simulink model "untitled1"  (R2014b)
settings: Solver=ode45  StartTime=0.0  StopTime=0.02  RelTol=1e-3
undefined symbols (not defined in the file or in its folder): powergui
libraries: powerlib x11
settings Model: Creator=JPSOLIV  LastModifiedBy=JPSOLIV

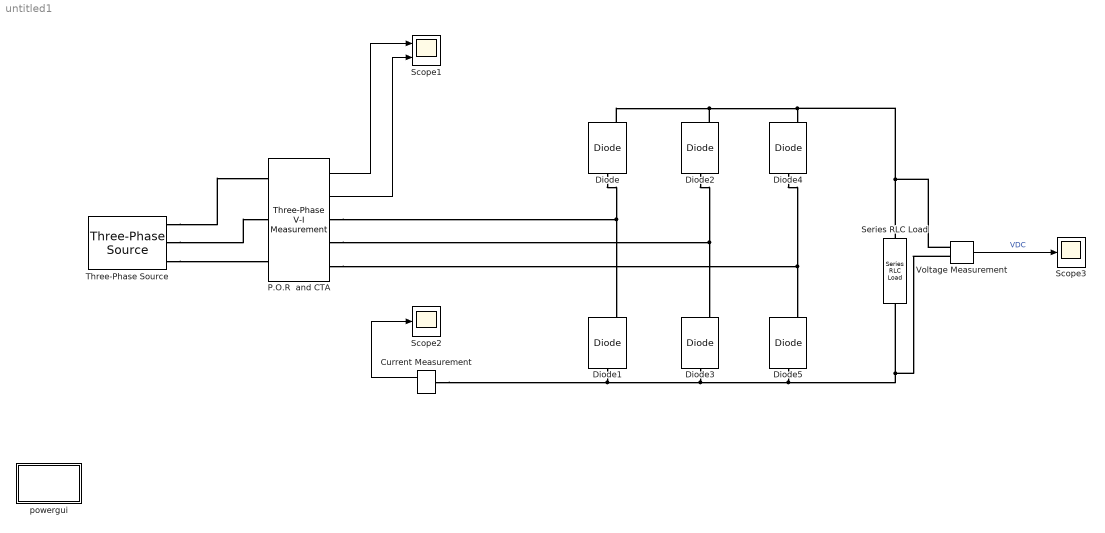
== system untitled1 ==
  Current Measurement : powerlib/Measurements/Current Measurement  PhasorSimulation=off  OutputType=Complex  PSBequivalent=0
  Diode{,1..5} (6 alike) : powerlib/Power Electronics/Diode  Ron=0.001  Lon=0  Vf=0.8  IC=0  UseSnubber=off  Rs=500  Cs=250e-9  Measurements=on
  P.O.R  and CTA : powerlib/Measurements/Three-Phase V-I Measurement  VoltageMeasurement=phase-to-phase  SetLabelV=off  LabelV=Vabc  Vpu=off  VpuLL=off  CurrentMeasurement=yes  SetLabelI=off  LabelI=Iabc  Ipu=off  Pbase=100e6  Vbase=500e3  OutputType=Complex  PhasorSimulation=off  PSBequivalent=0
  Scope1 : Scope  NumInputPorts=2
      settings: TimeRange=0.005  YMin=-200~-5  YMax=200~5  Decimation=100  SampleTime=1e-3
  Scope2 : Scope
      settings: TimeRange=0.005  YMin=-200  YMax=200  Decimation=100  SampleTime=1e-3
  Scope3 : Scope
      settings: TimeRange=0.005  YMin=-200  YMax=200  SaveName=ScopeData2  Decimation=100  SampleTime=1e-3
  Series RLC Load : powerlib/Elements/Series RLC Load  LConnTagsString=a  RConnTagsString=__new0  NominalVoltage=280  NominalFrequency=400  ActivePower=200  InductivePower=100  CapacitivePower=0  Setx0=off  InitialVoltage=0  SetiL0=off  InitialCurrent=0  Measurements=None
  Three-Phase Source : powerlib/Electrical Sources/Three-Phase Source  Voltage=115*sqrt(3)  PhaseAngle=0  Frequency=400  InternalConnection=Yn  SpecifyImpedance=off  Resistance=0.8929e-6  Inductance=16.58e-3*1e-6  ShortCircuitLevel=100e6  BaseVoltage=25e3  XRratio=7  BusType=swing  Pref=0  Qref=0  Qmin=-inf  Qmax=inf
  Voltage Measurement : powerlib/Measurements/Voltage Measurement  PhasorSimulation=off  OutputType=Complex  PSBequivalent=0
  powergui : Subsystem  Priority=1  AncestorBlock=powerlib/powergui  InitFcn=powergui( 'InitFcn_Callback' , gcb , 0 , [ ] );  StopFcn=powergui( 'StopFcn_Callback' , gcb , 0 , [ ] );  mask(PSB option menu block){SimulationMode=Discrete, SolverType=Tustin, SampleTime=1e-7, frequency=60, SPID=off, DisableSnubberDevices=off, DisableRonSwitches=off, DisableVfSwitches=off, SwTol=0, DisplayEquations=off, Interpol=off, methode=off, Ts=0, frequencyindice=0, Pbase=100e6, ErrMax=1e-4, Iterations=50, UnitsV=kV, UnitsW=MW, FunctionMessages=off, echomessages=off, HookPort=off, EnableUseOfTLC=off, x0status=blocks, RestoreLinks=warning, ResistiveCurrentMeasurement=off, Frange=[0:2:500], Ylog=off, Xlog=on, ShowGrid=off, save=off, variable=ZData, structure=0, ZoomFFT=off, StartTime=0.0, cycles=1, DisplayStyle=1, fundamental=60, FreqAxis=off, MaxFrequency=1000, frequencyindicesteady=1, RmsSteady=1, display=off}
      mask prompts: SimulationMode "Simulation type:"; SolverType "Solver type:"; SampleTime "Sample time (s):"; frequency "Phasor frequency (Hz):"; SPID "Enable use of ideal switching devices"; DisableSnubberDevices "Disable snubbers in switching devices"; DisableRonSwitches "Disable On resistance in switching devices (Ron=0)"; DisableVfSwitches "Disable Forward voltage in switching devices (Vf=0)"; SwTol "Switch tolerance"; DisplayEquations "Display circuit differential equations"; Interpol "Interpolate"; methode "Store state-space matrices"; Ts "Buffer size (MBytes)"; frequencyindice "Load flow frequency (Hz):"; Pbase "Base power Pbase (VA):"; ErrMax "PQ tolerance (pu):"; Iterations "Max iterations:"; UnitsV "Voltage units"; UnitsW "Power units"; FunctionMessages "Disable SimPowerSystems warnings"; echomessages "Display SimPowerSystems compilation messages"; HookPort "Add a hook port to the powergui block"; EnableUseOfTLC "Use TLC file when in Accelerator Simulation Mode and for code generation"; x0status "Start simulation with initial electrical states from:"; RestoreLinks "Restore disabled links of SimPowerSystems blocks:"; ResistiveCurrentMeasurement "Use non ideal current measurement blocks (1e-4Ohm internal resistance)"; Frange "Frequency Range"; Ylog "Log impedance"; Xlog "log Frequency"; ShowGrid "grid"; save "Save Data To Workspace"; variable "Variable Name"; structure "Structure Name (PSBFFTSCOPE)"; ZoomFFT "ZoomFFT (PSBFFTSCOPE)"; StartTime "Start Time (PSBFFTSCOPE)"; cycles "Cycles (PSBFFTSCOPE)"; DisplayStyle "Display style (PSBFFTSCOPE)"; fundamental "Fundamental (PSBFFTSCOPE)"; FreqAxis "Frequency Axis (PSBFFTSCOPE)"; MaxFrequency "Max Frequency (PSBFFTSCOPE)"; frequencyindicesteady "Frequency indice (STEADYSTATE)"; RmsSteady "RMS display (STEADYSTATE)"; display "Display Results"
      mask help: Set simulation type, simulation parameters, and preferences
      mask init:
      | message = powergui('MaskInitialization',gcb,SimulationMode,SampleTime);
      settings: CopyFcn=powergui( 'Copy_Callback' , gcb , 0 , [ ] );  ModelCloseFcn=powergui( 'CloseButton_Callback' , gcb , [ ] , [ ] );  NameChangeFcn=powergui( 'NameChangeFcn_Callback' , gcb , 0 , [ ] );  OpenFcn=powergui(gcb,'Open')
      settings: DeleteFcn=|
      | % see geck 675031 powergui( 'Copy_Callback' , gcb , 1 , [ ] );
      | 
      | powergui( 'CloseButton_Callback' , gcb , [ ] , [ ] );
      settings: PreSaveFcn=|
      | powergui( 'PreSaveFcn_Callback' , gcb , [ ] , [ ] );
      | powergui( 'CloseButton_Callback' , gcb , [ ] , [ ] );
      mask Help: helpview(psbhelp)
      mask TypeOptions SimulationMode: Continuous | Discrete | Phasor
      mask Callback SimulationMode: powergui('SimulationType',[],[],gcb);
      mask TypeOptions SolverType: Tustin/Backward Euler (TBE) | Tustin | Backward Euler
      mask Callback SolverType: powergui('SolverType',[],[],gcb);
      mask Callback SPID: powergui('SPID',[],[],gcb);
      mask Callback Interpol: powergui('INTERPOLATE',[],[],gcb);
      mask Callback methode: powergui('STORE',[],[],gcb);
      mask TypeOptions UnitsV: V | kV
      mask TypeOptions UnitsW: W | kW | MW
      mask Callback HookPort: powergui('HookPort',[],[],gcb);
      mask TypeOptions x0status: blocks | steady | zero
      mask TypeOptions RestoreLinks: yes | warning | no
      mask DialogControl Advanced Prompt: Advanced settings (Tustin solver)
      mask Display: color('blue'),disp(message)
  wires:
  Voltage Measurement/1 -> Scope3/1  "VDC"
  P.O.R  and CTA/1 -> Scope1/1
  P.O.R  and CTA/2 -> Scope1/2
  Current Measurement/1 -> Scope2/1
  connections:
  Diode/LConn1 -- P.O.R  and CTA/RConn1 -- Diode1/RConn1
  Diode2/LConn1 -- P.O.R  and CTA/RConn2 -- Diode3/RConn1
  Diode4/RConn1 -- Diode/RConn1 -- Diode2/RConn1 -- Series RLC Load/LConn1 -- Voltage Measurement/LConn1
  Voltage Measurement/LConn2 -- Series RLC Load/RConn1 -- Diode5/LConn1 -- Current Measurement/LConn1 -- Diode1/LConn1 -- Diode3/LConn1
  Diode4/LConn1 -- P.O.R  and CTA/RConn3 -- Diode5/RConn1
  Three-Phase Source/RConn1 -- P.O.R  and CTA/LConn1
  Three-Phase Source/RConn2 -- P.O.R  and CTA/LConn2
  Three-Phase Source/RConn3 -- P.O.R  and CTA/LConn3

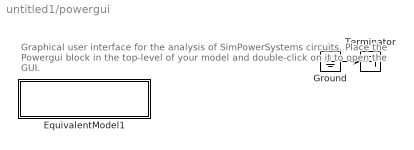
== system untitled1/powergui ==
  note: Graphical user interface for the analysis of  SimPowerSystems circuits.
      | Place the Powergui block in the top-level of your model and double-click
      | on it to open the GUI.
  EquivalentModel1 : Subsystem
      mask init:
      | S  = GetDataForEquivalentModel('Discrete',gcbh);
      mask Display:
      | color('red')
      | disp('EQUIVALENT CIRCUIT\nDiscrete')
  Ground : Ground
  Terminator : Terminator
  wires:
  Ground/1 -> Terminator/1

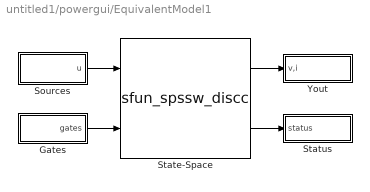
== system untitled1/powergui/EquivalentModel1 ==
  Gates : Subsystem
  Sources : Subsystem
  State-Space : S-Function  FunctionName=sfun_spssw_discc  Parameters=S.Ts,S.A, S.B, S.C, S.D, S.x0, S.EnableUseOfTLC,S.SwitchResistance ,S.SwitchType, S.SwitchGateInitialValue, S.OutputsToResetToZero, S.TBEON  EnableBusSupport=off
  Status : Subsystem
  Yout : Subsystem
  wires:
  State-Space/1 -> Yout/1(v,i)
  State-Space/2 -> Status/1(status)
  Sources/1(u) -> State-Space/1
  Gates/1(gates) -> State-Space/2

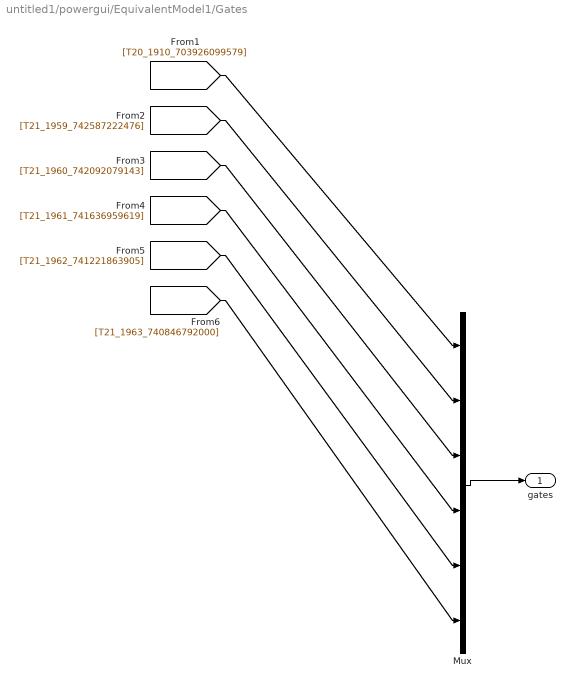
== system untitled1/powergui/EquivalentModel1/Gates ==
  Mux : Mux  Inputs=[1 1 1 1 1 1]
  gates : Outport
  wires:
  Mux/1 -> gates/1
  [T20_1910_703926099579] -> Mux/1
  [T21_1959_742587222476] -> Mux/2
  [T21_1960_742092079143] -> Mux/3
  [T21_1961_741636959619] -> Mux/4
  [T21_1962_741221863905] -> Mux/5
  [T21_1963_740846792000] -> Mux/6

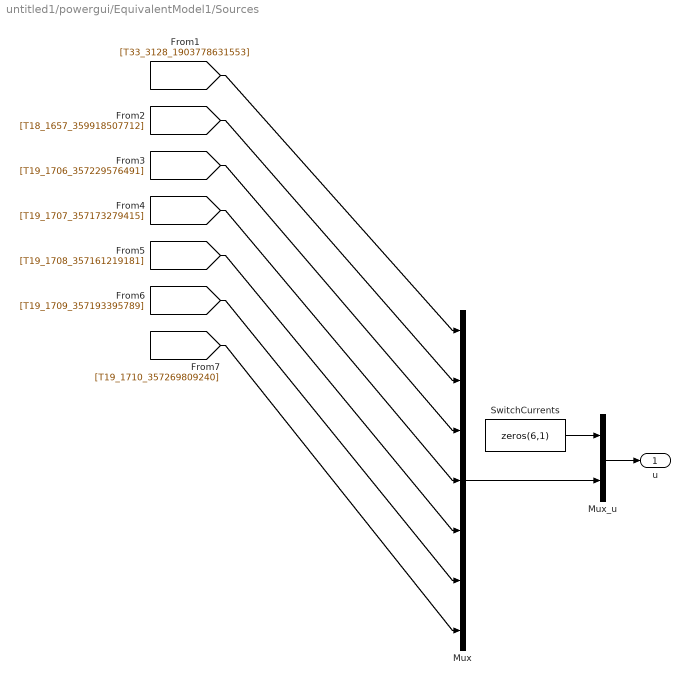
== system untitled1/powergui/EquivalentModel1/Sources ==
  Mux : Mux  Inputs=[3 1 1 1 1 1 1]
  Mux_u : Mux  Inputs=[6 9]
  SwitchCurrents : Constant  Value=zeros(6,1)
  u : Outport
  wires:
  Mux/1 -> Mux_u/2
  SwitchCurrents/1 -> Mux_u/1
  Mux_u/1 -> u/1
  [T33_3128_1903778631553] -> Mux/1
  [T18_1657_359918507712] -> Mux/2
  [T19_1706_357229576491] -> Mux/3
  [T19_1707_357173279415] -> Mux/4
  [T19_1708_357161219181] -> Mux/5
  [T19_1709_357193395789] -> Mux/6
  [T19_1710_357269809240] -> Mux/7

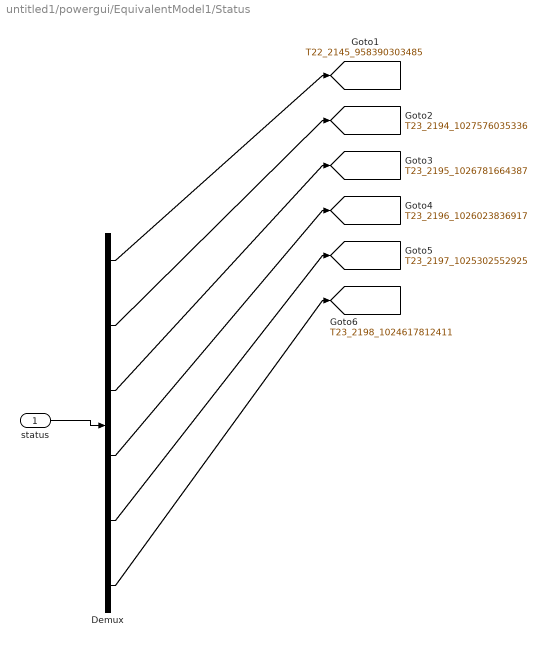
== system untitled1/powergui/EquivalentModel1/Status ==
  status : Inport
  Demux : Demux  Outputs=[1 1 1 1 1 1]
  tag scope: T22_2145_958390303485=global, T23_2194_1027576035336=global, T23_2195_1026781664387=global, T23_2196_1026023836917=global, T23_2197_1025302552925=global, T23_2198_1024617812411=global
  wires:
  status/1 -> Demux/1
  Demux/1 -> [T22_2145_958390303485]
  Demux/2 -> [T23_2194_1027576035336]
  Demux/3 -> [T23_2195_1026781664387]
  Demux/4 -> [T23_2196_1026023836917]
  Demux/5 -> [T23_2197_1025302552925]
  Demux/6 -> [T23_2198_1024617812411]

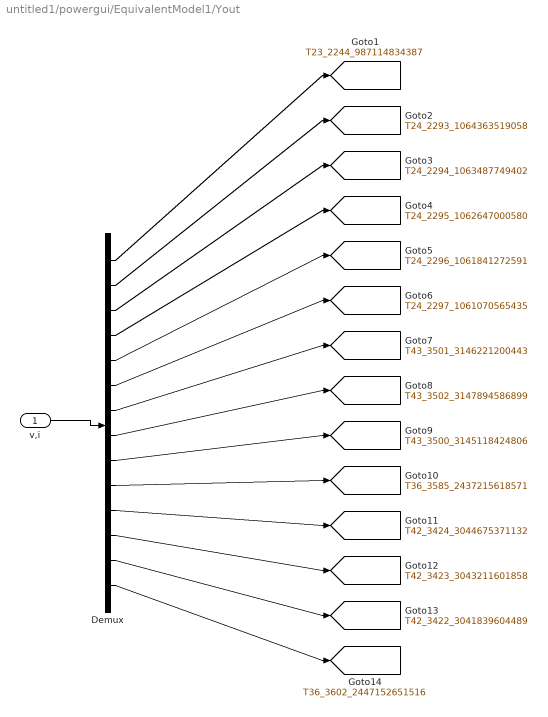
== system untitled1/powergui/EquivalentModel1/Yout ==
  v,i : Inport
  Demux : Demux  Outputs=[1 1 1 1 1 1 1 1 1 1 1 1 1 1]
  tag scope: T23_2244_987114834387=global, T24_2293_1064363519058=global, T24_2294_1063487749402=global, T24_2295_1062647000580=global, T24_2296_1061841272591=global, T24_2297_1061070565435=global, T36_3585_2437215618571=global, T36_3602_2447152651516=global, T42_3422_3041839604489=global, T42_3423_3043211601858=global, T42_3424_3044675371132=global, T43_3500_3145118424806=global, T43_3501_3146221200443=global, T43_3502_3147894586899=global
  wires:
  v,i/1 -> Demux/1
  Demux/1 -> [T23_2244_987114834387]
  Demux/2 -> [T24_2293_1064363519058]
  Demux/3 -> [T24_2294_1063487749402]
  Demux/4 -> [T24_2295_1062647000580]
  Demux/5 -> [T24_2296_1061841272591]
  Demux/6 -> [T24_2297_1061070565435]
  Demux/7 -> [T43_3501_3146221200443]
  Demux/8 -> [T43_3502_3147894586899]
  Demux/9 -> [T43_3500_3145118424806]
  Demux/10 -> [T36_3585_2437215618571]
  Demux/11 -> [T42_3424_3044675371132]
  Demux/12 -> [T42_3423_3043211601858]
  Demux/13 -> [T42_3422_3041839604489]
  Demux/14 -> [T36_3602_2447152651516]
